simulink model "Motor_Position_Control"  (R2020a)
settings: Solver=VariableStepAuto  StartTime=0.0  StopTime=10  RelTol=1e-3
PreLoadFcn:
  | L = 2.75E-6;
  | R = 4;
  | b = 3.5077E-6;
  | J = 3.2284E-6;
  | K = 0.0274;
settings Model: DataDictionary=Dictionary_Problem4.sldd  Creator=Admin  LastModifiedBy=Admin
settings DataIOCC: SaveOutput=off  SaveTime=off

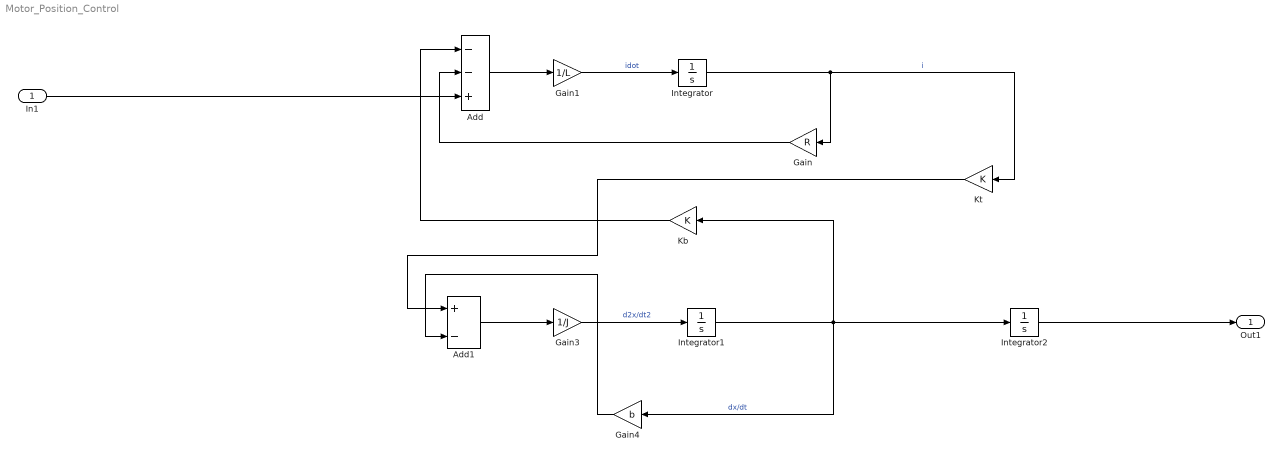
== system Motor_Position_Control ==
  In1 : Inport  OutDataTypeStr=double  PortDimensions=1  SampleTime=0
  Add : Sum  Inputs=--+
  Add1 : Sum  Inputs=+-
  Gain : Gain  Gain=R
  Gain1 : Gain  Gain=1/L
  Gain3 : Gain  Gain=1/J
  Gain4 : Gain  Gain=b
  Integrator : Integrator
  Integrator1 : Integrator
  Integrator2 : Integrator
  Kb : Gain  Gain=K
  Kt : Gain  Gain=K
  Out1 : Outport  OutDataTypeStr=double  PortDimensions=1  SampleTime=0
  wires:
  Add1/1 -> Gain3/1
  Gain1/1 -> Integrator/1  "idot"
  Add/1 -> Gain1/1
  Integrator1/1 -> Gain4/1, Kb/1, Integrator2/1  "dx/dt"
  Gain3/1 -> Integrator1/1  "d2x/dt2"
  Kb/1 -> Add/1
  Gain4/1 -> Add1/2
  Kt/1 -> Add1/1
  Gain/1 -> Add/2
  Integrator/1 -> Kt/1, Gain/1  "i"
  Integrator2/1 -> Out1/1
  In1/1 -> Add/3
